simulink model "regt"  (R2023a)
settings: Solver=FixedStepDiscrete  StartTime=0.0  StopTime=10.0  FixedStep=0.01  MaxStep=0.001  RelTol=1e-3
settings Model: Creator=mrrom  LastModifiedBy=mrrom
settings DataIOCC: SaveOutput=off  SaveTime=off

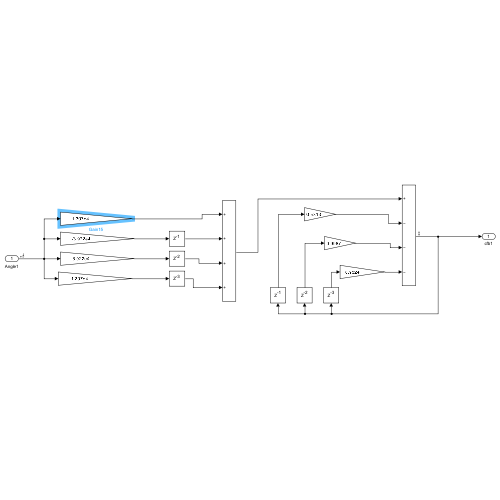
[thumbnail: Simulink's stored preview of the top-level diagram]
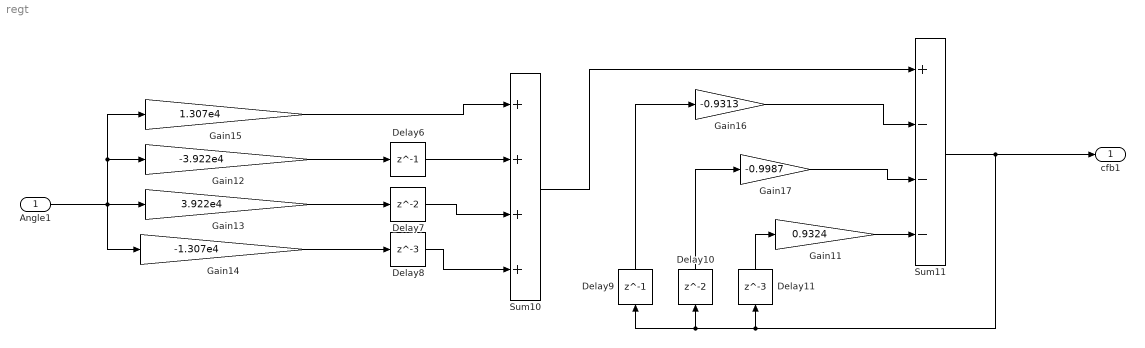
== system regt ==
  Angle1 : Inport  OutDataTypeStr=double  PortDimensions=1  SampleTime=[0.01,0]
  Delay10 : Delay  SampleTime=0.01
  Delay11 : Delay  DelayLength=3  SampleTime=0.01
  Delay6 : Delay  DelayLength=1  SampleTime=0.01
  Delay7 : Delay  SampleTime=0.01
  Delay8 : Delay  DelayLength=3  SampleTime=0.01
  Delay9 : Delay  DelayLength=1  SampleTime=0.01
  Gain11 : Gain  Gain=0.9324
  Gain12 : Gain  Gain=-3.922e4
  Gain13 : Gain  Gain=3.922e4
  Gain14 : Gain  Gain=-1.307e4
  Gain15 : Gain  Gain=1.307e4
  Gain16 : Gain  Gain=-0.9313
  Gain17 : Gain  Gain=-0.9987
  Sum10 : Sum  Inputs=++++
  Sum11 : Sum  Inputs=+---
  cfb1 : Outport  OutDataTypeStr=double  PortDimensions=1  SampleTime=[0.01,0]
  wires:
  Sum11/1 -> Delay10/1, Delay9/1, Delay11/1, cfb1/1
  Gain17/1 -> Sum11/3
  Gain11/1 -> Sum11/4
  Delay11/1 -> Gain11/1
  Delay8/1 -> Sum10/4
  Delay6/1 -> Sum10/2
  Gain15/1 -> Sum10/1
  Angle1/1 -> Gain15/1, Gain12/1, Gain14/1, Gain13/1
  Delay7/1 -> Sum10/3
  Gain12/1 -> Delay6/1
  Delay9/1 -> Gain16/1
  Delay10/1 -> Gain17/1
  Gain16/1 -> Sum11/2
  Gain13/1 -> Delay7/1
  Gain14/1 -> Delay8/1
  Sum10/1 -> Sum11/1
